simulink model "nonlinearLIM"  (R2021b)
settings: Solver=VariableStepAuto  StartTime=0.0  StopTime=10.0  RelTol=1e-3
settings Model: Creator=Ferran  LastModifiedBy=Ferran

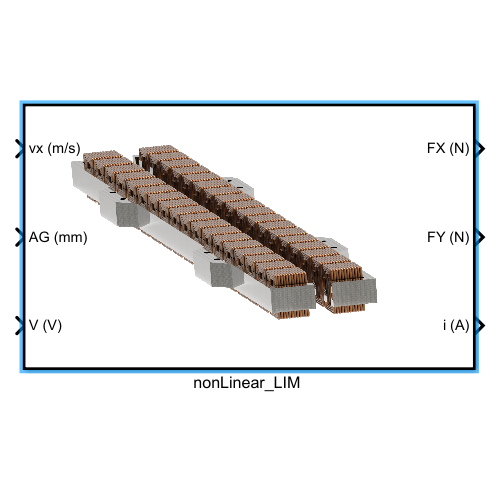
[thumbnail: Simulink's stored preview of the top-level diagram]
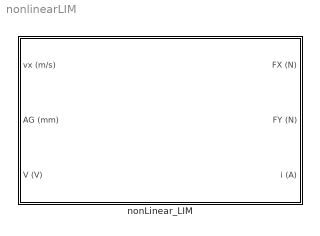
== system nonlinearLIM ==
  "nonLinear_LIM " : Subsystem  TreatAsAtomicUnit=on
      mask Display: image('$imagefile'); % Use "Edit Image" on toolstrip to change.

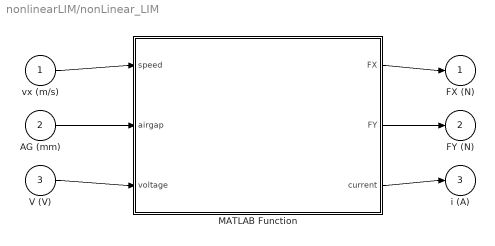
== system nonlinearLIM/nonLinear_LIM  ==
  vx (m/s) : Inport
  AG (mm) : Inport  Port=2
  V (V) : Inport  Port=3
  MATLAB Function : MATLAB Function  TreatAsAtomicUnit=on
  FX (N) : Outport
  FY (N) : Outport  Port=2
  i (A) : Outport  Port=3
  wires:
  MATLAB Function/1(FX) -> FX (N)/1
  MATLAB Function/2(FY) -> FY (N)/1
  MATLAB Function/3(current) -> i (A)/1
  AG (mm)/1 -> MATLAB Function/2(airgap)
  vx (m/s)/1 -> MATLAB Function/1(speed)
  V (V)/1 -> MATLAB Function/3(voltage)

== matlab function nonlinearLIM/nonLinear_LIM /MATLAB Function ==
  data: speed input; FX output; airgap input; voltage input; FY output; current output; pod parameter
function [FX, FY, current] = nonlinearLIM(speed, airgap, voltage, pod)
% Computes the forces (traction and transversal, both in N) and the current
% consumed by the motor, as a function of speed (m/s), airgap (mm) and
% voltage (V)
% ═════════════════════════════════════════════════════════════════════════
% Last updated: 03.02.2022
% ═════════════════════════════════════════════════════════════════════════

x1 = speed;
x2 = airgap;
x3 = voltage;

FX = pod.propulsion.x.p10 * x3 +  pod.propulsion.x.p11 * x1 * x3;

current = pod.propulsion.current.p00 + pod.propulsion.current.p10*x3 + ...
          pod.propulsion.current.p01*x1 + pod.propulsion.current.p11*x3*x1 +...
          pod.propulsion.current.p02*x1^2;

FY = 1.7514.*x3 - 2.4586.*x2 - 0.41812.*x2.*x3 + 0.6979.*x2.^2 + ...
     0.015655.*x2.^2.*x3 -2.3696.*x1 + 0.041473.*x1.*x3 + ...
     0.19953.*x1.*x2 - 0.016205.*x1.*x2.*x3 + 0.078832.*x1.*x2.^2 + ...
     0.51065.*x1.^2 + 0.0048345.*x1.^2.*x3 -0.10518.*x1.^2.*x2 + ...
     4.3394.*1 -0.0075967.*x1.^3-0.084085.*x2.^3;
